simulink model "EGRVlv_VDPosGov"  (R2016b)
settings: configuration reference "CodeGenConfigSet" (kept outside this file)
values from neighbouring files (symbols this model uses):
  EGRVlv_ctClnUpFin_C = Calibration.Parameter    [init_EGRVlv_VDPosGov.m]
  EGRVlv_DKdNgv_C = Calibration.Parameter    [init_EGRVlv_VDPosGov.m]
  EGRVlv_DKdPsv_C = Calibration.Parameter    [init_EGRVlv_VDPosGov.m]
  EGRVlv_drActNgv_C = Calibration.Parameter    [init_EGRVlv_VDPosGov.m]
  EGRVlv_facCrntEffFlt_C = Calibration.Parameter    [init_EGRVlv_VDPosGov.m]
  EGRVlv_iEff_CUR = Calibration.Parameter    [init_EGRVlv_VDPosGov.m]
  EGRVlv_iEff_CURX = Calibration.Parameter    [init_EGRVlv_VDPosGov.m]
  EGRVlv_iEffOvrLd_C = Calibration.Parameter    [init_EGRVlv_VDPosGov.m]
  EGRVlv_IKiLMSSlp_C = Calibration.Parameter    [init_EGRVlv_VDPosGov.m]
  EGRVlv_IKiNgv_C = Calibration.Parameter    [init_EGRVlv_VDPosGov.m]
  EGRVlv_IKiPsv_C = Calibration.Parameter    [init_EGRVlv_VDPosGov.m]
  EGRVlv_KdParDT1_C = Calibration.Parameter    [init_EGRVlv_VDPosGov.m]
  EGRVlv_PKpNgv_C = Calibration.Parameter    [init_EGRVlv_VDPosGov.m]
  EGRVlv_PKpPsv_C = Calibration.Parameter    [init_EGRVlv_VDPosGov.m]
  EGRVlv_rActNgv_C = Calibration.Parameter    [init_EGRVlv_VDPosGov.m]
  EGRVlv_rDesClnUpCls_C = Calibration.Parameter    [init_EGRVlv_VDPosGov.m]
  EGRVlv_rDesClnUpOpen_C = Calibration.Parameter    [init_EGRVlv_VDPosGov.m]
  EGRVlv_rDesEGR_CUR = Calibration.Parameter    [init_EGRVlv_VDPosGov.m]
  EGRVlv_rDesEGR_CURX = Calibration.Parameter    [init_EGRVlv_VDPosGov.m]
  EGRVlv_rDesLMSMin_C = Calibration.Parameter    [init_EGRVlv_VDPosGov.m]
  EGRVlv_rDesOffHold_C = Calibration.Parameter    [init_EGRVlv_VDPosGov.m]
  EGRVlv_rEGRDflVal_C = Calibration.Parameter    [init_EGRVlv_VDPosGov.m]
  EGRVlv_rEGRSwtOff_C = Calibration.Parameter    [init_EGRVlv_VDPosGov.m]
  EGRVlv_rGovDvtThres_C = Calibration.Parameter    [init_EGRVlv_VDPosGov.m]
  EGRVlv_rGovMax_C = Calibration.Parameter    [init_EGRVlv_VDPosGov.m]
  EGRVlv_rGovMax_CUR = Calibration.Parameter    [init_EGRVlv_VDPosGov.m]
  EGRVlv_rGovMax_CURX = Calibration.Parameter    [init_EGRVlv_VDPosGov.m]
  EGRVlv_rGovMin_C = Calibration.Parameter    [init_EGRVlv_VDPosGov.m]
  EGRVlv_rGovMin_CUR = Calibration.Parameter    [init_EGRVlv_VDPosGov.m]
  EGRVlv_rGovMin_CURX = Calibration.Parameter    [init_EGRVlv_VDPosGov.m]
  EGRVlv_rIniStp_C = Calibration.Parameter    [init_EGRVlv_VDPosGov.m]
  EGRVlv_rOutDMax_C = Calibration.Parameter    [init_EGRVlv_VDPosGov.m]
  EGRVlv_rOutIMax_C = Calibration.Parameter    [init_EGRVlv_VDPosGov.m]
  EGRVlv_rPIDWinNgv_C = Calibration.Parameter    [init_EGRVlv_VDPosGov.m]
  EGRVlv_rPIDWinPsv_C = Calibration.Parameter    [init_EGRVlv_VDPosGov.m]
  EGRVlv_rSwtOffRmp_C = Calibration.Parameter    [init_EGRVlv_VDPosGov.m]
  EGRVlv_SlwClsDKd_C = Calibration.Parameter    [init_EGRVlv_VDPosGov.m]
  EGRVlv_SlwClsIKi_C = Calibration.Parameter    [init_EGRVlv_VDPosGov.m]
  EGRVlv_SlwClsPKp_C = Calibration.Parameter    [init_EGRVlv_VDPosGov.m]
  EGRVlv_SmlSigNgvDKd_C = Calibration.Parameter    [init_EGRVlv_VDPosGov.m]
  EGRVlv_SmlSigNgvIKi_C = Calibration.Parameter    [init_EGRVlv_VDPosGov.m]
  EGRVlv_SmlSigNgvPKp_C = Calibration.Parameter    [init_EGRVlv_VDPosGov.m]
  EGRVlv_SmlSigPsvDKd_C = Calibration.Parameter    [init_EGRVlv_VDPosGov.m]
  EGRVlv_SmlSigPsvIKi_C = Calibration.Parameter    [init_EGRVlv_VDPosGov.m]
  EGRVlv_SmlSigPsvPKp_C = Calibration.Parameter    [init_EGRVlv_VDPosGov.m]
  EGRVLV_STCLNUP_CLOSE = fi(3,State_uint8)    [init_EGRVlv_VDPosGov.m]
  EGRVLV_STCLNUP_FINISH = fi(4,State_uint8)    [init_EGRVlv_VDPosGov.m]
  EGRVLV_STCLNUP_INIT = fi(1,State_uint8)    [init_EGRVlv_VDPosGov.m]
  EGRVLV_STCLNUP_OPEN = fi(2,State_uint8)    [init_EGRVlv_VDPosGov.m]
  EGRVlv_stClnUpInh_C = Calibration.Parameter    [init_EGRVlv_VDPosGov.m]
  EGRVlv_swtDesValNrmInv_C = Calibration.Parameter    [init_EGRVlv_VDPosGov.m]
  EGRVlv_swtEGRTyp_C = Calibration.Parameter    [init_EGRVlv_VDPosGov.m]
  EGRVlv_swtGovByp_C = Calibration.Parameter    [init_EGRVlv_VDPosGov.m]
  EGRVlv_swtSelDT1In_C = Calibration.Parameter    [init_EGRVlv_VDPosGov.m]
  EGRVlv_tiClnUp_C = Calibration.Parameter    [init_EGRVlv_VDPosGov.m]
  EGRVlv_tiGovDT1_C = Calibration.Parameter    [init_EGRVlv_VDPosGov.m]
  EGRVlv_tiLimDlyOvrLd_C = Calibration.Parameter    [init_EGRVlv_VDPosGov.m]
  EGRVlv_tiOutIMax_C = Calibration.Parameter    [init_EGRVlv_VDPosGov.m]
  EGRVlv_tiParDT1_C = Calibration.Parameter    [init_EGRVlv_VDPosGov.m]
  MINUS_1_PRC = fi(-1,Prc_100_rate)    [init_EGRVlv_VDPosGov.m]
  RLS = fi(0,State_uint8)    [init_EGRVlv_VDPosGov.m]
  VALEO = fi(0,State_uint8)    [init_EGRVlv_VDPosGov.m]
  ZERO_PRC = fi(0,Prc_100_rate)    [init_EGRVlv_VDPosGov.m]
undefined symbols (not defined in the file or in its folder): CEngDsT_tTransf_CURX, EGRVlv_VDPosGov_DT, SubSysExeState_conv
libraries: CXLib x32, simulink x12
(part 1 of 2)
settings Model: Creator=lvzhanghui  LastModifiedBy=zhoutinglin
settings ConfigSetRef: SourceLocation=Base Workspace

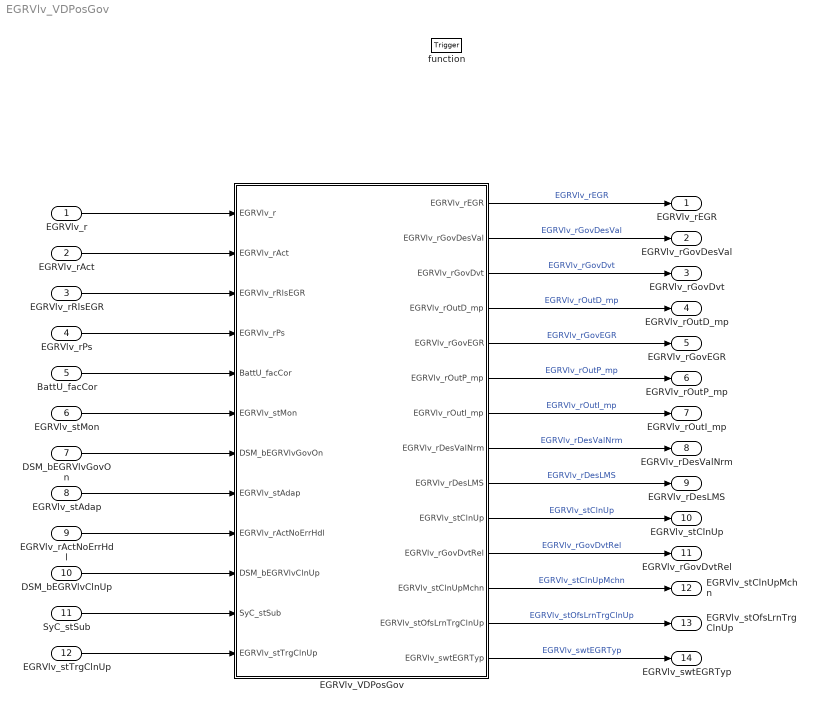
== system EGRVlv_VDPosGov ==
  EGRVlv_r : Inport  Tag=%  Description=Commanded value from application SW  OutMin=-100  OutMax=100  OutDataTypeStr=Prc_100_rate
  EGRVlv_rAct : Inport  Tag=%  Description=Actuatorposition  Port=2  OutMin=-100  OutMax=100  OutDataTypeStr=Prc_100_rate
  EGRVlv_rRlsEGR : Inport  Tag=%  Description=Additional control value to release a jammed valve  Port=3  OutMin=-100  OutMax=100  OutDataTypeStr=Prc_100_rate
  EGRVlv_rPs : Inport  Tag=%  Description=Duty cycle to power stage  Port=4  OutMin=-100  OutMax=100  OutDataTypeStr=Prc_100_rate
  BattU_facCor : Inport  Description=Battery correction factor  Port=5  OutMin=-32  OutMax=31.9  OutDataTypeStr=Factor
  EGRVlv_stMon : Inport  Description=State of system monitoring  Port=6  OutMin=0  OutMax=65535  OutDataTypeStr=State_uint16
  DSM_bEGRVlvGovOn : Inport  Description=Status of FId_EGRVlvGovOn  Port=7  OutMin=0  OutMax=1  OutDataTypeStr=boolean
  EGRVlv_stAdap : Inport  Description=Status of offset learning  Port=8  OutMin=0  OutMax=65535  OutDataTypeStr=State_uint16
  EGRVlv_rActNoErrHdl : Inport  Tag=%  Description=Valve position (offset corrected without error handling)  Port=9  OutMin=-100  OutMax=100  OutDataTypeStr=Prc_100_rate
  DSM_bEGRVlvClnUp : Inport  Description=Status of FId_EGRVlvClnUp  Port=10  OutMin=0  OutMax=1  OutDataTypeStr=boolean
  SyC_stSub : Inport  Description=Current system/ECU sub-state  Port=11  OutDataTypeStr=Enum: SubSysExeState_conv
  EGRVlv_stTrgClnUp : Inport  Description=Status of valve cleaning trigger, in case of unsuccessful offset learning because of plausibility errors  Port=12  OutMin=0  OutMax=1  OutDataTypeStr=boolean
  function : TriggerPort  TriggerType=function-call  VariantControl=Variant
  EGRVlv_VDPosGov : Subsystem
  EGRVlv_rEGR : Outport  Tag=%  Description=Control value for the EGR valve  OutMin=-100  OutMax=100  OutDataTypeStr=Prc_100_rate
  EGRVlv_rGovDesVal : Outport  Tag=%  Description=Internal desired value for governor  Port=2  OutMin=-100  OutMax=100  OutDataTypeStr=Prc_100_rate
  EGRVlv_rGovDvt : Outport  Tag=%  Description=Control deviation  Port=3  OutMin=-100  OutMax=100  OutDataTypeStr=Prc_100_rate
  EGRVlv_rOutD_mp : Outport  Tag=%  Description=measurement point for D governor for single flow implementation  Port=4  OutMin=-100  OutMax=100  OutDataTypeStr=Prc_100_rate
  EGRVlv_rGovEGR : Outport  Tag=%  Description=Control value from the governor  Port=5  OutMin=-100  OutMax=100  OutDataTypeStr=Prc_100_rate
  EGRVlv_rOutP_mp : Outport  Tag=%  Description=measurement point for P governor for single flow implementation  Port=6  OutMin=-100  OutMax=100  OutDataTypeStr=Prc_100_rate
  EGRVlv_rOutI_mp : Outport  Tag=%  Description=measurement point for I governor for single flow implementation  Port=7  OutMin=-100  OutMax=100  OutDataTypeStr=Prc_100_rate
  EGRVlv_rDesValNrm : Outport  Tag=%  Description=Normalized desired value  Port=8  OutMin=-100  OutMax=100  OutDataTypeStr=Prc_100_rate
  EGRVlv_rDesLMS : Outport  Tag=%  Description=Desired value from LMS control  Port=9  OutMin=-100  OutMax=100  OutDataTypeStr=Prc_100_rate
  EGRVlv_stClnUp : Outport  Description=Status of valvle cleanup function  Port=10  OutMin=0  OutMax=255  OutDataTypeStr=State_uint8
  EGRVlv_rGovDvtRel : Outport  Tag=%  Description=Relative governor deviation for OBD purpose  Port=11  OutMin=-100  OutMax=100  OutDataTypeStr=Prc_100_rate
  EGRVlv_stClnUpMchn : Outport  Description=Status of cleanup state machine  Port=12  OutMin=0  OutMax=255  OutDataTypeStr=State_uint8
  EGRVlv_stOfsLrnTrgClnUp : Outport  Description=Offset learning trigger from EGR valve cleanup function  Port=13  OutMin=0  OutMax=1  OutDataTypeStr=boolean
  EGRVlv_swtEGRTyp : Outport  Description=Type of EGR actuator used  Port=14  OutMin=0  OutMax=255  OutDataTypeStr=State_uint8
  wires:
  EGRVlv_r/1 -> EGRVlv_VDPosGov/1(EGRVlv_r)
  EGRVlv_rAct/1 -> EGRVlv_VDPosGov/2(EGRVlv_rAct)
  EGRVlv_rRlsEGR/1 -> EGRVlv_VDPosGov/3(EGRVlv_rRlsEGR)
  EGRVlv_rPs/1 -> EGRVlv_VDPosGov/4(EGRVlv_rPs)
  BattU_facCor/1 -> EGRVlv_VDPosGov/5(BattU_facCor)
  EGRVlv_stMon/1 -> EGRVlv_VDPosGov/6(EGRVlv_stMon)
  DSM_bEGRVlvGovOn/1 -> EGRVlv_VDPosGov/7(DSM_bEGRVlvGovOn)
  EGRVlv_stAdap/1 -> EGRVlv_VDPosGov/8(EGRVlv_stAdap)
  EGRVlv_rActNoErrHdl/1 -> EGRVlv_VDPosGov/9(EGRVlv_rActNoErrHdl)
  DSM_bEGRVlvClnUp/1 -> EGRVlv_VDPosGov/10(DSM_bEGRVlvClnUp)
  SyC_stSub/1 -> EGRVlv_VDPosGov/11(SyC_stSub)
  EGRVlv_stTrgClnUp/1 -> EGRVlv_VDPosGov/12(EGRVlv_stTrgClnUp)
  EGRVlv_VDPosGov/1(EGRVlv_rEGR) -> EGRVlv_rEGR/1  "EGRVlv_rEGR"
  EGRVlv_VDPosGov/2(EGRVlv_rGovDesVal) -> EGRVlv_rGovDesVal/1  "EGRVlv_rGovDesVal"
  EGRVlv_VDPosGov/3(EGRVlv_rGovDvt) -> EGRVlv_rGovDvt/1  "EGRVlv_rGovDvt"
  EGRVlv_VDPosGov/4(EGRVlv_rOutD_mp) -> EGRVlv_rOutD_mp/1  "EGRVlv_rOutD_mp"
  EGRVlv_VDPosGov/5(EGRVlv_rGovEGR) -> EGRVlv_rGovEGR/1  "EGRVlv_rGovEGR"
  EGRVlv_VDPosGov/6(EGRVlv_rOutP_mp) -> EGRVlv_rOutP_mp/1  "EGRVlv_rOutP_mp"
  EGRVlv_VDPosGov/7(EGRVlv_rOutI_mp) -> EGRVlv_rOutI_mp/1  "EGRVlv_rOutI_mp"
  EGRVlv_VDPosGov/8(EGRVlv_rDesValNrm) -> EGRVlv_rDesValNrm/1  "EGRVlv_rDesValNrm"
  EGRVlv_VDPosGov/9(EGRVlv_rDesLMS) -> EGRVlv_rDesLMS/1  "EGRVlv_rDesLMS"
  EGRVlv_VDPosGov/10(EGRVlv_stClnUp) -> EGRVlv_stClnUp/1  "EGRVlv_stClnUp"
  EGRVlv_VDPosGov/11(EGRVlv_rGovDvtRel) -> EGRVlv_rGovDvtRel/1  "EGRVlv_rGovDvtRel"
  EGRVlv_VDPosGov/12(EGRVlv_stClnUpMchn) -> EGRVlv_stClnUpMchn/1  "EGRVlv_stClnUpMchn"
  EGRVlv_VDPosGov/13(EGRVlv_stOfsLrnTrgClnUp) -> EGRVlv_stOfsLrnTrgClnUp/1  "EGRVlv_stOfsLrnTrgClnUp"
  EGRVlv_VDPosGov/14(EGRVlv_swtEGRTyp) -> EGRVlv_swtEGRTyp/1  "EGRVlv_swtEGRTyp"

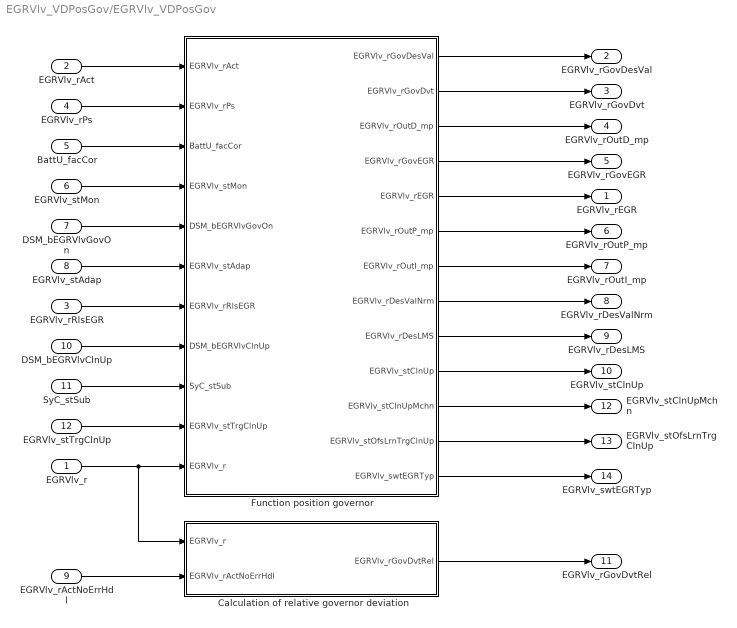
== system EGRVlv_VDPosGov/EGRVlv_VDPosGov ==
  EGRVlv_r : Inport  Tag=%
  EGRVlv_rAct : Inport  Tag=%  Port=2
  EGRVlv_rRlsEGR : Inport  Tag=%  Port=3
  EGRVlv_rPs : Inport  Tag=%  Port=4
  BattU_facCor : Inport  Port=5
  EGRVlv_stMon : Inport  Port=6
  DSM_bEGRVlvGovOn : Inport  Port=7
  EGRVlv_stAdap : Inport  Port=8
  EGRVlv_rActNoErrHdl : Inport  Tag=%  Port=9
  DSM_bEGRVlvClnUp : Inport  Tag=%  Port=10
  SyC_stSub : Inport  Tag=%  Port=11
  EGRVlv_stTrgClnUp : Inport  Tag=%  Port=12
  Calculation of relative governor deviation : Subsystem
  Function position governor : Subsystem
  EGRVlv_rEGR : Outport  Tag=%
  EGRVlv_rGovDesVal : Outport  Tag=%  Port=2
  EGRVlv_rGovDvt : Outport  Tag=%  Port=3
  EGRVlv_rOutD_mp : Outport  Tag=%  Port=4
  EGRVlv_rGovEGR : Outport  Tag=%  Port=5
  EGRVlv_rOutP_mp : Outport  Tag=%  Port=6
  EGRVlv_rOutI_mp : Outport  Tag=%  Port=7
  EGRVlv_rDesValNrm : Outport  Tag=%  Port=8
  EGRVlv_rDesLMS : Outport  Tag=%  Port=9
  EGRVlv_stClnUp : Outport  Port=10
  EGRVlv_rGovDvtRel : Outport  Tag=%  Port=11
  EGRVlv_stClnUpMchn : Outport  Tag=%  Port=12
  EGRVlv_stOfsLrnTrgClnUp : Outport  Tag=%  Port=13
  EGRVlv_swtEGRTyp : Outport  Tag=%  Port=14
  wires:
  EGRVlv_r/1 -> Function position governor/11(EGRVlv_r), Calculation of relative governor deviation/1(EGRVlv_r)
  EGRVlv_rActNoErrHdl/1 -> Calculation of relative governor deviation/2(EGRVlv_rActNoErrHdl)
  EGRVlv_rAct/1 -> Function position governor/1(EGRVlv_rAct)
  EGRVlv_rPs/1 -> Function position governor/2(EGRVlv_rPs)
  BattU_facCor/1 -> Function position governor/3(BattU_facCor)
  EGRVlv_stMon/1 -> Function position governor/4(EGRVlv_stMon)
  DSM_bEGRVlvGovOn/1 -> Function position governor/5(DSM_bEGRVlvGovOn)
  EGRVlv_stAdap/1 -> Function position governor/6(EGRVlv_stAdap)
  EGRVlv_rRlsEGR/1 -> Function position governor/7(EGRVlv_rRlsEGR)
  DSM_bEGRVlvClnUp/1 -> Function position governor/8(DSM_bEGRVlvClnUp)
  SyC_stSub/1 -> Function position governor/9(SyC_stSub)
  EGRVlv_stTrgClnUp/1 -> Function position governor/10(EGRVlv_stTrgClnUp)
  Calculation of relative governor deviation/1(EGRVlv_rGovDvtRel) -> EGRVlv_rGovDvtRel/1
  Function position governor/1(EGRVlv_rGovDesVal) -> EGRVlv_rGovDesVal/1
  Function position governor/2(EGRVlv_rGovDvt) -> EGRVlv_rGovDvt/1
  Function position governor/3(EGRVlv_rOutD_mp) -> EGRVlv_rOutD_mp/1
  Function position governor/4(EGRVlv_rGovEGR) -> EGRVlv_rGovEGR/1
  Function position governor/5(EGRVlv_rEGR) -> EGRVlv_rEGR/1
  Function position governor/6(EGRVlv_rOutP_mp) -> EGRVlv_rOutP_mp/1
  Function position governor/7(EGRVlv_rOutI_mp) -> EGRVlv_rOutI_mp/1
  Function position governor/8(EGRVlv_rDesValNrm) -> EGRVlv_rDesValNrm/1
  Function position governor/9(EGRVlv_rDesLMS) -> EGRVlv_rDesLMS/1
  Function position governor/10(EGRVlv_stClnUp) -> EGRVlv_stClnUp/1
  Function position governor/11(EGRVlv_stClnUpMchn) -> EGRVlv_stClnUpMchn/1
  Function position governor/12(EGRVlv_stOfsLrnTrgClnUp) -> EGRVlv_stOfsLrnTrgClnUp/1
  Function position governor/13(EGRVlv_swtEGRTyp) -> EGRVlv_swtEGRTyp/1

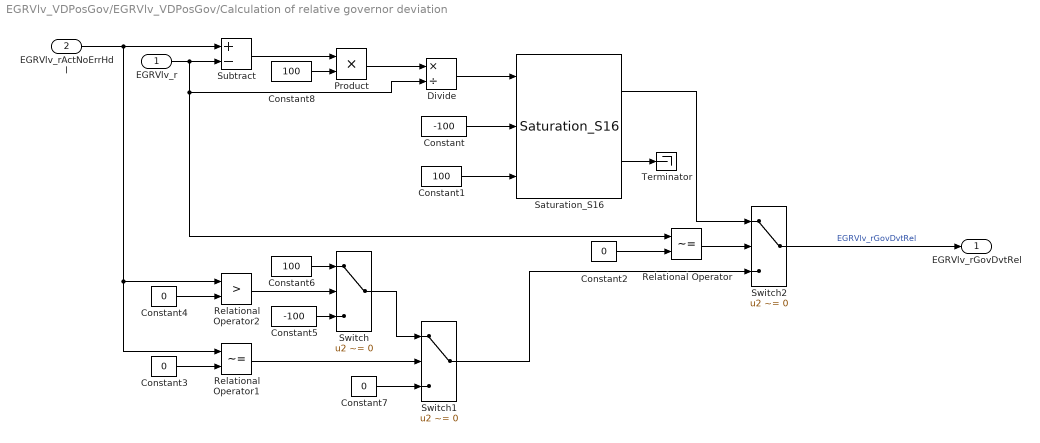
== system EGRVlv_VDPosGov/EGRVlv_VDPosGov/Calculation of relative governor deviation ==
  EGRVlv_r : Inport  Tag=%
  EGRVlv_rActNoErrHdl : Inport  Tag=%  Port=2
  Constant : Constant  Value=-100  OutDataTypeStr=Prc_100_rate
  Constant1 : Constant  Value=100  OutDataTypeStr=Prc_100_rate
  Constant2 : Constant  Value=0  OutDataTypeStr=Inherit: Inherit via back propagation
  Constant3 : Constant  Value=0  OutDataTypeStr=Inherit: Inherit via back propagation
  Constant4 : Constant  Value=0  OutDataTypeStr=Inherit: Inherit via back propagation
  Constant5 : Constant  Value=-100  OutDataTypeStr=Prc_100_rate
  Constant6 : Constant  Value=100  OutDataTypeStr=Prc_100_rate
  Constant7 : Constant  Value=0  OutDataTypeStr=Prc_100_rate
  Constant8 : Constant  Value=100  OutDataTypeStr=uint8
  Divide : Product  Inputs=*/  OutDataTypeStr=Prc_100_rate  SaturateOnIntegerOverflow=on
  Product : Product  OutDataTypeStr=fixdt(1,16,10000/8192,0)  SaturateOnIntegerOverflow=on
  Relational Operator : RelationalOperator  Operator=~=  OutDataTypeStr=boolean  RndMeth=Simplest  InputSameDT=on
  Relational Operator1 : RelationalOperator  Operator=~=  OutDataTypeStr=boolean  RndMeth=Simplest  InputSameDT=on
  Relational Operator2 : RelationalOperator  Operator=>  OutDataTypeStr=boolean  RndMeth=Simplest  InputSameDT=on
  Saturation_S16 : CXLib/Saturation_S16
  Subtract : Sum  Inputs=+-  SaturateOnIntegerOverflow=on
  Switch : Switch  Criteria=u2 ~= 0
  Switch1 : Switch  Criteria=u2 ~= 0
  Switch2 : Switch  Criteria=u2 ~= 0
  Terminator : Terminator
  EGRVlv_rGovDvtRel : Outport  Tag=%
  wires:
  EGRVlv_r/1 -> Relational Operator/1, Divide/2, Subtract/2
  Subtract/1 -> Product/1
  Product/1 -> Divide/1
  Divide/1 -> Saturation_S16/1
  Constant/1 -> Saturation_S16/2
  Constant1/1 -> Saturation_S16/3
  Constant2/1 -> Relational Operator/2
  EGRVlv_rActNoErrHdl/1 -> Subtract/1, Relational Operator1/1, Relational Operator2/1
  Constant3/1 -> Relational Operator1/2
  Constant4/1 -> Relational Operator2/2
  Relational Operator2/1 -> Switch/2
  Constant6/1 -> Switch/1
  Constant5/1 -> Switch/3
  Switch/1 -> Switch1/1
  Constant7/1 -> Switch1/3
  Relational Operator1/1 -> Switch1/2
  Relational Operator/1 -> Switch2/2
  Switch1/1 -> Switch2/3
  Saturation_S16/1 -> Switch2/1
  Switch2/1 -> EGRVlv_rGovDvtRel/1  "EGRVlv_rGovDvtRel"
  Constant8/1 -> Product/2
  Saturation_S16/2 -> Terminator/1

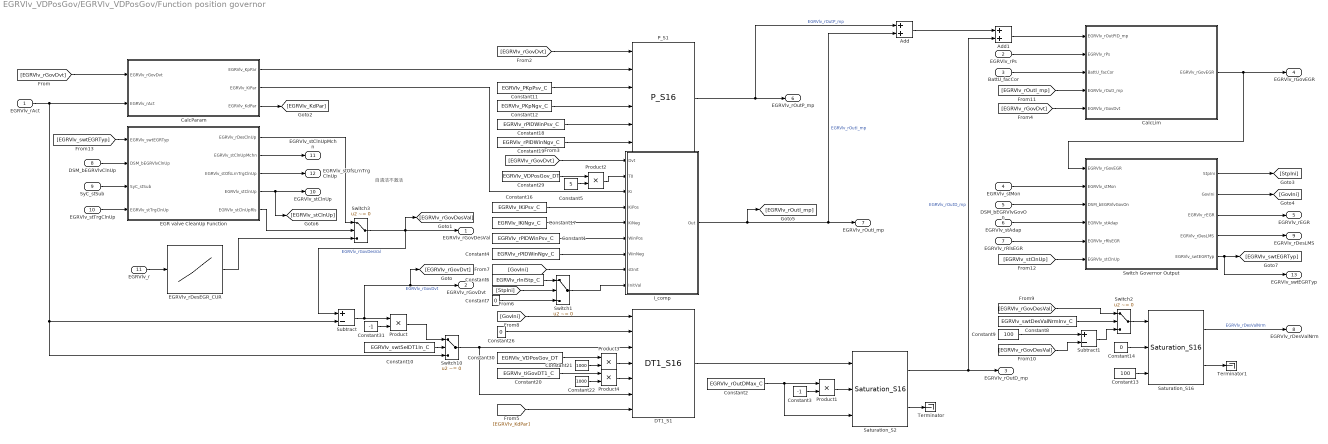
== system EGRVlv_VDPosGov/EGRVlv_VDPosGov/Function position governor ==
  note: 自清洁不激活
  EGRVlv_rAct : Inport  Tag=%
  EGRVlv_rPs : Inport  Tag=%  Port=2
  BattU_facCor : Inport  Tag=%  Port=3
  EGRVlv_stMon : Inport  Tag=%  Port=4
  DSM_bEGRVlvGovOn : Inport  Tag=%  Port=5
  EGRVlv_stAdap : Inport  Tag=%  Port=6
  EGRVlv_rRlsEGR : Inport  Tag=%  Port=7
  DSM_bEGRVlvClnUp : Inport  Tag=%  Port=8
  SyC_stSub : Inport  Tag=%  Port=9
  EGRVlv_stTrgClnUp : Inport  Tag=%  Port=10
  EGRVlv_r : Inport  Tag=%  Port=11
  Add : Sum  SaturateOnIntegerOverflow=on
  Add1 : Sum  SaturateOnIntegerOverflow=on
  CalcLim : Subsystem
  CalcParam : Subsystem
  Constant1 : Constant  Value=EGRVlv_rPIDWinPsv_C
  Constant10 : Constant  Value=EGRVlv_swtSelDT1In_C
  Constant11 : Constant  Value=EGRVlv_PKpPsv_C
  Constant12 : Constant  Value=EGRVlv_PKpNgv_C
  Constant13 : Constant  Value=100  OutDataTypeStr=Prc_100_rate
  Constant14 : Constant  Value=0  OutDataTypeStr=Prc_100_rate
  Constant16 : Constant  Value=EGRVlv_IKiPsv_C
  Constant17 : Constant  Value=EGRVlv_IKiNgv_C
  Constant18 : Constant  Value=EGRVlv_rPIDWinPsv_C
  Constant19 : Constant  Value=EGRVlv_rPIDWinNgv_C
  Constant2 : Constant  Value=EGRVlv_rOutDMax_C
  Constant20 : Constant  Value=EGRVlv_tiGovDT1_C
  Constant21 : Constant  Value=1000  OutDataTypeStr=uint16
  Constant22 : Constant  Value=1000  OutDataTypeStr=uint16
  Constant26 : Constant  Value=0  OutDataTypeStr=Inherit: Inherit via back propagation
  Constant29 : Constant  Value=EGRVlv_VDPosGov_DT
  Constant3 : Constant  Value=-1  OutDataTypeStr=int8
  Constant30 : Constant  Value=EGRVlv_VDPosGov_DT
  Constant31 : Constant  Value=-1  OutDataTypeStr=int8
  Constant4 : Constant  Value=EGRVlv_rPIDWinNgv_C
  Constant5 : Constant  Value=5  OutDataTypeStr=uint32
  Constant6 : Constant  Value=EGRVlv_rIniStp_C
  Constant7 : Constant  Value=0  OutDataTypeStr=Inherit: Inherit via back propagation
  Constant8 : Constant  Value=EGRVlv_swtDesValNrmInv_C
  Constant9 : Constant  Value=100  OutDataTypeStr=Prc_100_rate
  DT1_S1 : CXLib/DT1_S16
  EGR valve CleanUp Function : Subsystem
  EGRVlv_rDesEGR_CUR : Lookup_n-D  DialogController=Simulink.DDGSource  NumberOfTableDimensions=1  BreakpointsForDimension1=EGRVlv_rDesEGR_CURX  BreakpointsForDimension2=CEngDsT_tTransf_CURX  IndexSearchMethod=Linear search  BeginIndexSearchUsingPreviousIndexResult=on  Table=EGRVlv_rDesEGR_CUR  TableDataTypeStr=Inherit: Inherit from 'Table data'  ExtrapMethod=Clip  UseLastTableValue=on  InternalRulePriority=Speed  OutDataTypeStr=Inherit: Inherit from 'Table data'  SaturateOnIntegerOverflow=on
  I_comp : Subsystem
  P_S1 : CXLib/P_S16
  Product : Product  OutDataTypeStr=Prc_100_rate  SaturateOnIntegerOverflow=on
  Product1 : Product  OutDataTypeStr=Prc_100_rate  SaturateOnIntegerOverflow=on
  Product2 : Product  OutDataTypeStr=Inherit: Inherit via back propagation  SaturateOnIntegerOverflow=on
  Product3 : Product  OutDataTypeStr=uint32  SaturateOnIntegerOverflow=on
  Product4 : Product  OutDataTypeStr=uint32  SaturateOnIntegerOverflow=on
  Saturation_S16 : CXLib/Saturation_S16
  Saturation_S2 : CXLib/Saturation_S16
  Subtract : Sum  Inputs=+-  SaturateOnIntegerOverflow=on
  Subtract1 : Sum  Inputs=+-  SaturateOnIntegerOverflow=on
  Switch Governor Output : Subsystem
  Switch{1..3,10} (4 alike) : Switch  Criteria=u2 ~= 0
  Terminator : Terminator
  Terminator1 : Terminator
  EGRVlv_rGovDesVal : Outport  Tag=%
  EGRVlv_rGovDvt : Outport  Tag=%  Port=2
  EGRVlv_rOutD_mp : Outport  Tag=%  Port=3
  EGRVlv_rGovEGR : Outport  Tag=%  Port=4
  EGRVlv_rEGR : Outport  Tag=%  Port=5
  EGRVlv_rOutP_mp : Outport  Tag=%  Port=6
  EGRVlv_rOutI_mp : Outport  Tag=%  Port=7
  EGRVlv_rDesValNrm : Outport  Tag=%  Port=8
  EGRVlv_rDesLMS : Outport  Tag=%  Port=9
  EGRVlv_stClnUp : Outport  Tag=%  Port=10
  EGRVlv_stClnUpMchn : Outport  Tag=%  Port=11
  EGRVlv_stOfsLrnTrgClnUp : Outport  Tag=%  Port=12
  EGRVlv_swtEGRTyp : Outport  Tag=%  Port=13
  wires:
  Constant7/1 -> Switch1/3
  Constant8/1 -> Switch2/2
  Constant9/1 -> Subtract1/1
  EGRVlv_r/1 -> EGRVlv_rDesEGR_CUR/1
  Switch3/1 -> [EGRVlv_rGovDesVal], EGRVlv_rGovDesVal/1, Subtract/1  "EGRVlv_rGovDesVal"
  EGRVlv_rAct/1 -> CalcParam/2(EGRVlv_rAct), Subtract/2, Switch10/3
  Switch10/1 -> DT1_S1/6, DT1_S1/3
  Constant26/1 -> DT1_S1/2
  Constant10/1 -> Switch10/2
  Subtract/1 -> EGRVlv_rGovDvt/1, [EGRVlv_rGovDvt], Product/1  "EGRVlv_rGovDvt"
  Constant31/1 -> Product/2
  Product/1 -> Switch10/1
  DT1_S1/1 -> Saturation_S2/1
  Constant2/1 -> Saturation_S2/3, Product1/1
  Constant3/1 -> Product1/2
  Product1/1 -> Saturation_S2/2
  Saturation_S2/1 -> EGRVlv_rOutD_mp/1, Add1/2  "EGRVlv_rOutD_mp"
  Add/1 -> Add1/1
  Add1/1 -> CalcLim/1(EGRVlv_rOutPID_mp)
  [StpIni] -> Switch1/2
  Constant6/1 -> Switch1/1
  [EGRVlv_rGovDesVal] -> Subtract1/2
  Subtract1/1 -> Switch2/3
  [EGRVlv_rGovDesVal] -> Switch2/1
  Switch1/1 -> I_comp/9(InitVal)
  Constant14/1 -> Saturation_S16/2
  Constant12/1 -> P_S1/4
  Constant1/1 -> I_comp/6(WinPos)
  P_S1/1 -> EGRVlv_rOutP_mp/1, Add/1  "EGRVlv_rOutP_mp"
  Constant4/1 -> I_comp/7(WinNeg)
  Constant11/1 -> P_S1/3
  Constant19/1 -> P_S1/6
  Constant16/1 -> I_comp/4(KiPos)
  CalcParam/1(EGRVlv_KpPar) -> P_S1/2
  Constant18/1 -> P_S1/5
  CalcParam/2(EGRVlv_KiPar) -> I_comp/3(Ki)
  Constant17/1 -> I_comp/5(KiNeg)
  I_comp/1(Out) -> EGRVlv_rOutI_mp/1, Add/2, [EGRVlv_rOutI_mp]  "EGRVlv_rOutI_mp"
  CalcLim/1(EGRVlv_rGovEGR) -> EGRVlv_rGovEGR/1, Switch Governor Output/1(EGRVlv_rGovEGR)
  Constant13/1 -> Saturation_S16/3
  Switch2/1 -> Saturation_S16/1
  EGRVlv_rDesEGR_CUR/1 -> Switch3/3
  EGR valve CleanUp Function/1(EGRVlv_rDesClnUp) -> Switch3/1
  Constant21/1 -> Product3/2
  Product3/1 -> DT1_S1/4
  Constant30/1 -> Product3/1
  Constant22/1 -> Product4/2
  Constant20/1 -> Product4/1
  Product4/1 -> DT1_S1/5
  Switch Governor Output/5(EGRVlv_swtEGRTyp) -> EGRVlv_swtEGRTyp/1, [EGRVlv_swtEGRTyp]
  EGR valve CleanUp Function/4(EGRVlv_stClnUp) -> [EGRVlv_stClnUp], EGRVlv_stClnUp/1
  EGR valve CleanUp Function/5(EGRVlv_stClnUpRls) -> Switch3/2
  EGRVlv_rPs/1 -> CalcLim/2(EGRVlv_rPs)
  BattU_facCor/1 -> CalcLim/3(BattU_facCor)
  [EGRVlv_rOutI_mp] -> CalcLim/4(EGRVlv_rOutI_mp)
  [EGRVlv_rGovDvt] -> CalcParam/1(EGRVlv_rGovDvt)
  [GovIni] -> DT1_S1/1
  [EGRVlv_KdPar] -> DT1_S1/7
  [EGRVlv_swtEGRTyp] -> EGR valve CleanUp Function/1(EGRVlv_swtEGRTyp)
  DSM_bEGRVlvClnUp/1 -> EGR valve CleanUp Function/2(DSM_bEGRVlvClnUp)
  SyC_stSub/1 -> EGR valve CleanUp Function/3(SyC_stSub)
  EGRVlv_stTrgClnUp/1 -> EGR valve CleanUp Function/4(EGRVlv_stTrgClnUp)
  [EGRVlv_rGovDvt] -> I_comp/1(Dvt)
  [GovIni] -> I_comp/8(stInit)
  [EGRVlv_rGovDvt] -> CalcLim/5(EGRVlv_rGovDvt)
  [EGRVlv_rGovDvt] -> P_S1/1
  EGRVlv_stMon/1 -> Switch Governor Output/2(EGRVlv_stMon)
  DSM_bEGRVlvGovOn/1 -> Switch Governor Output/3(DSM_bEGRVlvGovOn)
  EGRVlv_stAdap/1 -> Switch Governor Output/4(EGRVlv_stAdap)
  EGRVlv_rRlsEGR/1 -> Switch Governor Output/5(EGRVlv_rRlsEGR)
  [EGRVlv_stClnUp] -> Switch Governor Output/6(EGRVlv_stClnUp)
  CalcParam/3(EGRVlv_KdPar) -> [EGRVlv_KdPar]
  EGR valve CleanUp Function/2(EGRVlv_stClnUpMchn) -> EGRVlv_stClnUpMchn/1
  EGR valve CleanUp Function/3(EGRVlv_stOfsLrnTrgClnUp) -> EGRVlv_stOfsLrnTrgClnUp/1
  Saturation_S16/1 -> EGRVlv_rDesValNrm/1  "EGRVlv_rDesValNrm"
  Saturation_S16/2 -> Terminator1/1
  Saturation_S2/2 -> Terminator/1
  Switch Governor Output/1(StpIni) -> [StpIni]
  Switch Governor Output/2(GovIni) -> [GovIni]
  Switch Governor Output/3(EGRVlv_rEGR) -> EGRVlv_rEGR/1
  Switch Governor Output/4(EGRVlv_rDesLMS) -> EGRVlv_rDesLMS/1
  Constant29/1 -> Product2/1
  Product2/1 -> I_comp/2(T0)
  Constant5/1 -> Product2/2

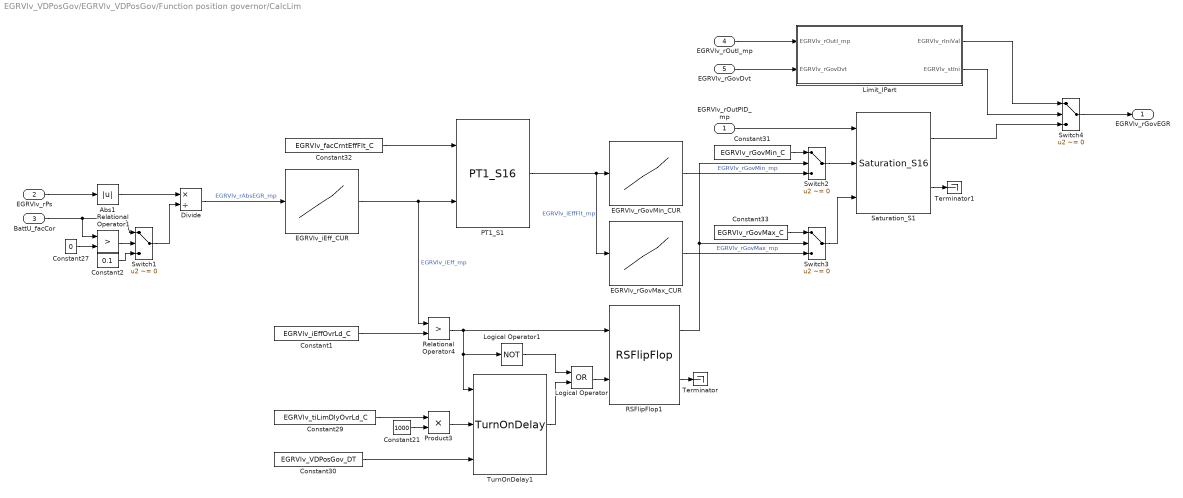
== system EGRVlv_VDPosGov/EGRVlv_VDPosGov/Function position governor/CalcLim ==
  EGRVlv_rOutPID_mp : Inport  Tag=%
  EGRVlv_rPs : Inport  Tag=%  Port=2
  BattU_facCor : Inport  Tag=%  Port=3
  EGRVlv_rOutI_mp : Inport  Tag=%  Port=4
  EGRVlv_rGovDvt : Inport  Tag=%  Port=5
  Abs1 : Abs
  Constant1 : Constant  Value=EGRVlv_iEffOvrLd_C
  Constant2 : Constant  Value=0.1  OutDataTypeStr=Inherit: Inherit via back propagation
  Constant21 : Constant  Value=1000  OutDataTypeStr=uint16
  Constant27 : Constant  Value=0  OutDataTypeStr=Inherit: Inherit via back propagation
  Constant29 : Constant  Value=EGRVlv_tiLimDlyOvrLd_C
  Constant30 : Constant  Value=EGRVlv_VDPosGov_DT
  Constant31 : Constant  Value=EGRVlv_rGovMin_C
  Constant32 : Constant  Value=EGRVlv_facCrntEffFlt_C
  Constant33 : Constant  Value=EGRVlv_rGovMax_C
  Divide : Product  Inputs=*/  OutDataTypeStr=Prc_100_rate  SaturateOnIntegerOverflow=on
  EGRVlv_iEff_CUR : Lookup_n-D  DialogController=Simulink.DDGSource  NumberOfTableDimensions=1  BreakpointsForDimension1=EGRVlv_iEff_CURX  BreakpointsForDimension2=CEngDsT_tTransf_CURX  IndexSearchMethod=Linear search  BeginIndexSearchUsingPreviousIndexResult=on  Table=EGRVlv_iEff_CUR  TableDataTypeStr=Inherit: Inherit from 'Table data'  ExtrapMethod=Clip  UseLastTableValue=on  InternalRulePriority=Speed  OutDataTypeStr=Inherit: Inherit from 'Table data'  SaturateOnIntegerOverflow=on
  EGRVlv_rGovMax_CUR : Lookup_n-D  DialogController=Simulink.DDGSource  NumberOfTableDimensions=1  BreakpointsForDimension1=EGRVlv_rGovMax_CURX  BreakpointsForDimension2=CEngDsT_tTransf_CURX  IndexSearchMethod=Linear search  BeginIndexSearchUsingPreviousIndexResult=on  Table=EGRVlv_rGovMax_CUR  TableDataTypeStr=Inherit: Inherit from 'Table data'  ExtrapMethod=Clip  UseLastTableValue=on  InternalRulePriority=Speed  OutDataTypeStr=Inherit: Inherit from 'Table data'  SaturateOnIntegerOverflow=on
  EGRVlv_rGovMin_CUR : Lookup_n-D  DialogController=Simulink.DDGSource  NumberOfTableDimensions=1  BreakpointsForDimension1=EGRVlv_rGovMin_CURX  BreakpointsForDimension2=CEngDsT_tTransf_CURX  IndexSearchMethod=Linear search  BeginIndexSearchUsingPreviousIndexResult=on  Table=EGRVlv_rGovMin_CUR  TableDataTypeStr=Inherit: Inherit from 'Table data'  ExtrapMethod=Clip  UseLastTableValue=on  InternalRulePriority=Speed  OutDataTypeStr=Inherit: Inherit from 'Table data'  SaturateOnIntegerOverflow=on
  Limit_IPart : Subsystem
  Logical Operator : Logic  Operator=OR  AllPortsSameDT=off  OutDataTypeStr=boolean
  Logical Operator1 : Logic  Operator=NOT  AllPortsSameDT=off  OutDataTypeStr=boolean
  PT1_S1 : CXLib/PT1_S16
  Product3 : Product  OutDataTypeStr=uint32  SaturateOnIntegerOverflow=on
  RSFlipFlop1 : CXLib/RSFlipFlop
  Relational Operator1 : RelationalOperator  Operator=>  OutDataTypeStr=boolean  RndMeth=Simplest  InputSameDT=on
  Relational Operator4 : RelationalOperator  Operator=>  OutDataTypeStr=boolean  RndMeth=Simplest
  Saturation_S1 : CXLib/Saturation_S16
  Switch{1..4} (4 alike) : Switch  Criteria=u2 ~= 0
  Terminator : Terminator
  Terminator1 : Terminator
  TurnOnDelay1 : CXLib/TurnOnDelay
  EGRVlv_rGovEGR : Outport  Tag=%
  wires:
  Abs1/1 -> Divide/1
  Constant33/1 -> Switch3/1
  RSFlipFlop1/1 -> Switch3/2, Switch2/2
  EGRVlv_rGovMax_CUR/1 -> Switch3/3  "EGRVlv_rGovMax_mp"
  Switch2/1 -> Saturation_S1/2
  Switch3/1 -> Saturation_S1/3
  TurnOnDelay1/1 -> Logical Operator/2
  Logical Operator/1 -> RSFlipFlop1/2
  Logical Operator1/1 -> Logical Operator/1
  Constant31/1 -> Switch2/1
  EGRVlv_iEff_CUR/1 -> PT1_S1/2, Relational Operator4/1  "EGRVlv_iEff_mp"
  EGRVlv_rGovMin_CUR/1 -> Switch2/3  "EGRVlv_rGovMin_mp"
  Constant1/1 -> Relational Operator4/2
  Relational Operator4/1 -> RSFlipFlop1/1, TurnOnDelay1/1, Logical Operator1/1
  EGRVlv_rPs/1 -> Abs1/1
  Divide/1 -> EGRVlv_iEff_CUR/1  "EGRVlv_rAbsEGR_mp"
  PT1_S1/1 -> EGRVlv_rGovMax_CUR/1, EGRVlv_rGovMin_CUR/1  "EGRVlv_iEffFlt_mp"
  Constant29/1 -> Product3/1
  Constant30/1 -> TurnOnDelay1/3
  BattU_facCor/1 -> Relational Operator1/1, Switch1/1
  Constant32/1 -> PT1_S1/1
  Relational Operator1/1 -> Switch1/2
  Constant27/1 -> Relational Operator1/2
  Constant2/1 -> Switch1/3
  Switch1/1 -> Divide/2
  Product3/1 -> TurnOnDelay1/2
  Limit_IPart/1(EGRVlv_rIniVal) -> Switch4/1
  Limit_IPart/2(EGRVlv_stIni) -> Switch4/2
  Switch4/1 -> EGRVlv_rGovEGR/1
  Saturation_S1/1 -> Switch4/3
  Constant21/1 -> Product3/2
  EGRVlv_rOutPID_mp/1 -> Saturation_S1/1
  RSFlipFlop1/2 -> Terminator/1
  Saturation_S1/2 -> Terminator1/1
  EGRVlv_rGovDvt/1 -> Limit_IPart/2(EGRVlv_rGovDvt)
  EGRVlv_rOutI_mp/1 -> Limit_IPart/1(EGRVlv_rOutI_mp)

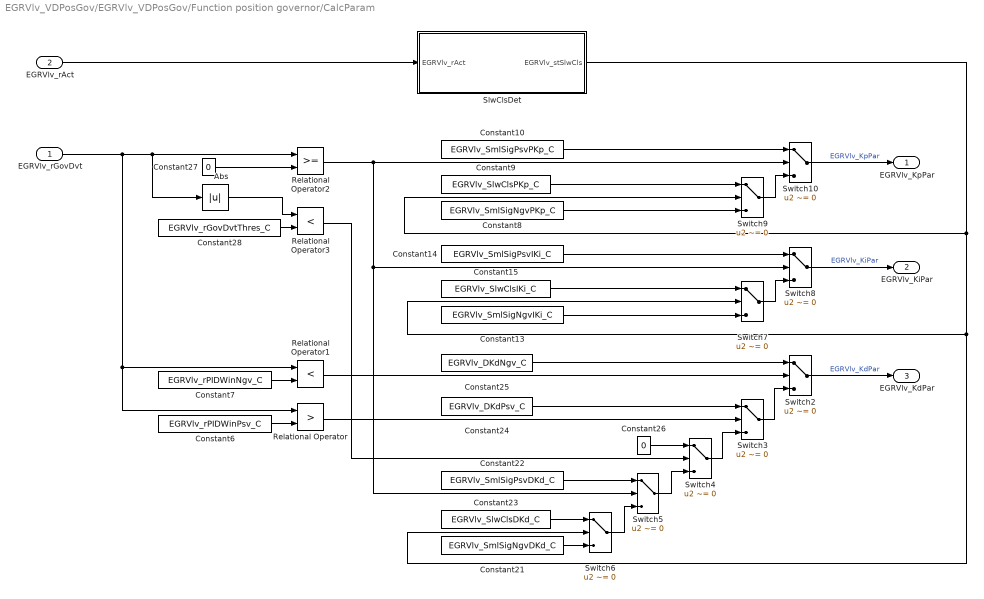
== system EGRVlv_VDPosGov/EGRVlv_VDPosGov/Function position governor/CalcParam ==
  EGRVlv_rGovDvt : Inport  Tag=%
  EGRVlv_rAct : Inport  Tag=%  Port=2
  Abs : Abs
  Constant10 : Constant  Value=EGRVlv_SmlSigPsvPKp_C
  Constant13 : Constant  Value=EGRVlv_SmlSigNgvIKi_C
  Constant14 : Constant  Value=EGRVlv_SmlSigPsvIKi_C
  Constant15 : Constant  Value=EGRVlv_SlwClsIKi_C
  Constant21 : Constant  Value=EGRVlv_SmlSigNgvDKd_C
  Constant22 : Constant  Value=EGRVlv_SmlSigPsvDKd_C
  Constant23 : Constant  Value=EGRVlv_SlwClsDKd_C
  Constant24 : Constant  Value=EGRVlv_DKdPsv_C
  Constant25 : Constant  Value=EGRVlv_DKdNgv_C
  Constant26 : Constant  Value=0  OutDataTypeStr=Inherit: Inherit via back propagation
  Constant27 : Constant  Value=0  OutDataTypeStr=Inherit: Inherit via back propagation
  Constant28 : Constant  Value=EGRVlv_rGovDvtThres_C
  Constant6 : Constant  Value=EGRVlv_rPIDWinPsv_C
  Constant7 : Constant  Value=EGRVlv_rPIDWinNgv_C
  Constant8 : Constant  Value=EGRVlv_SmlSigNgvPKp_C
  Constant9 : Constant  Value=EGRVlv_SlwClsPKp_C
  Relational Operator : RelationalOperator  Operator=>  OutDataTypeStr=boolean  RndMeth=Simplest
  Relational Operator1 : RelationalOperator  Operator=<  OutDataTypeStr=boolean  RndMeth=Simplest
  Relational Operator2 : RelationalOperator  OutDataTypeStr=boolean  RndMeth=Simplest  InputSameDT=on
  Relational Operator3 : RelationalOperator  Operator=<  OutDataTypeStr=boolean  RndMeth=Simplest
  SlwClsDet : Subsystem
  Switch{2..10} (9 alike) : Switch  Criteria=u2 ~= 0
  EGRVlv_KpPar : Outport  Tag=%
  EGRVlv_KiPar : Outport  Tag=%  Port=2
  EGRVlv_KdPar : Outport  Tag=%  Port=3
  wires:
  Constant6/1 -> Relational Operator/2
  EGRVlv_rGovDvt/1 -> Relational Operator2/1, Abs/1, Relational Operator1/1, Relational Operator/1
  Constant7/1 -> Relational Operator1/2
  Abs/1 -> Relational Operator3/1
  Constant27/1 -> Relational Operator2/2
  Constant28/1 -> Relational Operator3/2
  Relational Operator1/1 -> Switch2/2
  Constant25/1 -> Switch2/1
  Switch3/1 -> Switch2/3
  Relational Operator/1 -> Switch3/2
  Constant24/1 -> Switch3/1
  Switch4/1 -> Switch3/3
  Relational Operator3/1 -> Switch4/2
  Constant26/1 -> Switch4/1
  Switch5/1 -> Switch4/3
  Relational Operator2/1 -> Switch10/2, Switch8/2, Switch5/2
  Constant22/1 -> Switch5/1
  Switch6/1 -> Switch5/3
  Constant23/1 -> Switch6/1
  Constant21/1 -> Switch6/3
  Switch7/1 -> Switch8/3
  Constant14/1 -> Switch8/1
  Constant15/1 -> Switch7/1
  Constant13/1 -> Switch7/3
  SlwClsDet/1(EGRVlv_stSlwCls) -> Switch6/2, Switch7/2, Switch9/2
  Switch9/1 -> Switch10/3
  Constant10/1 -> Switch10/1
  Constant9/1 -> Switch9/1
  Constant8/1 -> Switch9/3
  Switch10/1 -> EGRVlv_KpPar/1  "EGRVlv_KpPar"
  Switch8/1 -> EGRVlv_KiPar/1  "EGRVlv_KiPar"
  Switch2/1 -> EGRVlv_KdPar/1  "EGRVlv_KdPar"
  EGRVlv_rAct/1 -> SlwClsDet/1(EGRVlv_rAct)

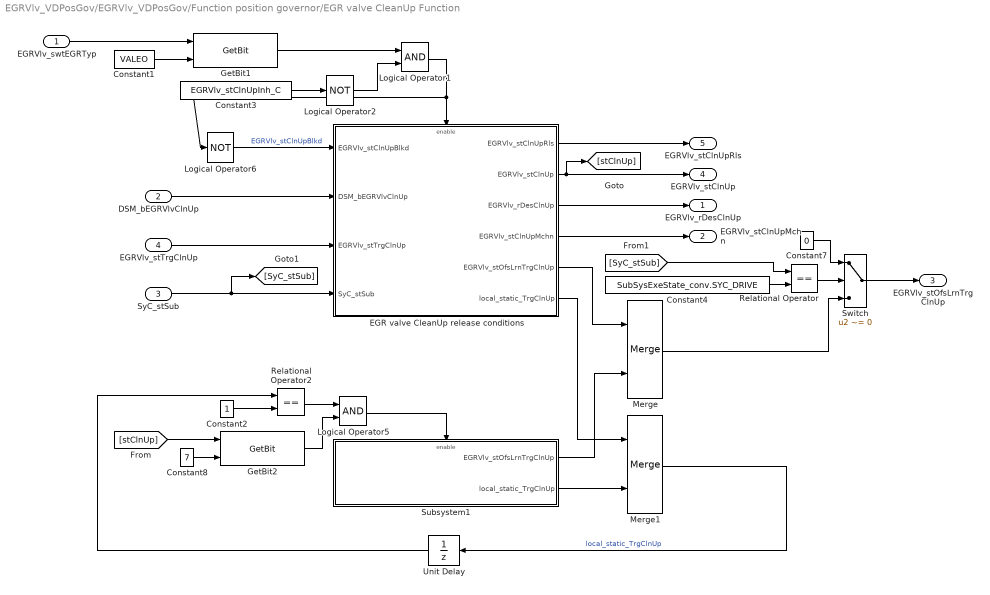
== system EGRVlv_VDPosGov/EGRVlv_VDPosGov/Function position governor/EGR valve CleanUp Function ==
  EGRVlv_swtEGRTyp : Inport  Tag=%
  DSM_bEGRVlvClnUp : Inport  Tag=%  Port=2
  SyC_stSub : Inport  Tag=%  Port=3
  EGRVlv_stTrgClnUp : Inport  Tag=%  Port=4
  Constant1 : Constant  Value=VALEO  OutDataTypeStr=uint8
  Constant2 : Constant  OutDataTypeStr=uint8
  Constant3 : Constant  Value=EGRVlv_stClnUpInh_C
  Constant4 : Constant  Value=SubSysExeState_conv.SYC_DRIVE  OutDataTypeStr=Enum:SubSysExeState_conv
  Constant7 : Constant  Value=0  OutDataTypeStr=boolean
  Constant8 : Constant  Value=7  OutDataTypeStr=uint8
  EGR valve CleanUp release conditions : Subsystem
  GetBit1 : CXLib/GetBit  dataTypeString=uint8  dataLength=0
      settings: AttributesFormatString=Get bit from %<dataTypeString>
  GetBit2 : CXLib/GetBit  dataTypeString=uint8  dataLength=0
      settings: AttributesFormatString=Get bit from %<dataTypeString>
  Logical Operator1 : Logic  AllPortsSameDT=off  OutDataTypeStr=boolean
  Logical Operator2 : Logic  Operator=NOT  AllPortsSameDT=off  OutDataTypeStr=boolean
  Logical Operator5 : Logic  AllPortsSameDT=off  OutDataTypeStr=boolean
  Logical Operator6 : Logic  Operator=NOT  AllPortsSameDT=off  OutDataTypeStr=boolean
  Merge : Merge
  Merge1 : Merge
  Relational Operator : RelationalOperator  Operator===  OutDataTypeStr=boolean  RndMeth=Simplest
  Relational Operator2 : RelationalOperator  Operator===  OutDataTypeStr=boolean  RndMeth=Simplest
  Subsystem1 : Subsystem
  Switch : Switch  Criteria=u2 ~= 0
  Unit Delay : UnitDelay  SampleTime=-1
      settings: AttributesFormatString=InitialValue=%<InitialCondition>
  EGRVlv_rDesClnUp : Outport  Tag=%
  EGRVlv_stClnUpMchn : Outport  Tag=%  Port=2
  EGRVlv_stOfsLrnTrgClnUp : Outport  Tag=%  Port=3
  EGRVlv_stClnUp : Outport  Tag=%  Port=4
  EGRVlv_stClnUpRls : Outport  Tag=%  Port=5
  wires:
  Constant1/1 -> GetBit1/2
  EGR valve CleanUp release conditions/6(local_static_TrgClnUp) -> Merge1/1
  Relational Operator2/1 -> Logical Operator5/1
  GetBit2/1 -> Logical Operator5/2
  Constant2/1 -> Relational Operator2/2
  Constant8/1 -> GetBit2/2
  EGR valve CleanUp release conditions/2(EGRVlv_stClnUp) -> [stClnUp], EGRVlv_stClnUp/1
  Merge1/1 -> Unit Delay/1  "local_static_TrgClnUp"
  Logical Operator5/1 -> Subsystem1/Enable
  Subsystem1/2(local_static_TrgClnUp) -> Merge1/2
  Subsystem1/1(EGRVlv_stOfsLrnTrgClnUp) -> Merge/2
  EGR valve CleanUp release conditions/5(EGRVlv_stOfsLrnTrgClnUp) -> Merge/1
  Unit Delay/1 -> Relational Operator2/1
  SyC_stSub/1 -> [SyC_stSub], EGR valve CleanUp release conditions/4(SyC_stSub)
  Logical Operator2/1 -> Logical Operator1/2
  Constant3/1 -> Logical Operator2/1
  GetBit1/1 -> Logical Operator1/1
  Logical Operator1/1 -> EGR valve CleanUp release conditions/Enable, Logical Operator6/1
  Constant4/1 -> Relational Operator/2
  Relational Operator/1 -> Switch/2
  Merge/1 -> Switch/3
  Switch/1 -> EGRVlv_stOfsLrnTrgClnUp/1
  Constant7/1 -> Switch/1
  [SyC_stSub] -> Relational Operator/1
  Logical Operator6/1 -> EGR valve CleanUp release conditions/1(EGRVlv_stClnUpBlkd)  "EGRVlv_stClnUpBlkd"
  DSM_bEGRVlvClnUp/1 -> EGR valve CleanUp release conditions/2(DSM_bEGRVlvClnUp)
  EGRVlv_stTrgClnUp/1 -> EGR valve CleanUp release conditions/3(EGRVlv_stTrgClnUp)
  EGRVlv_swtEGRTyp/1 -> GetBit1/1
  [stClnUp] -> GetBit2/1
  EGR valve CleanUp release conditions/1(EGRVlv_stClnUpRls) -> EGRVlv_stClnUpRls/1
  EGR valve CleanUp release conditions/3(EGRVlv_rDesClnUp) -> EGRVlv_rDesClnUp/1
  EGR valve CleanUp release conditions/4(EGRVlv_stClnUpMchn) -> EGRVlv_stClnUpMchn/1

== system EGRVlv_VDPosGov/EGRVlv_VDPosGov/Function position governor/I_comp ==
  note: %sampletime(us)%
  note: %1/s,resolution=2^15%
  Dvt : Inport
  T0 : Inport  Port=2  OutDataTypeStr=uint32
  Ki : Inport  Port=3
  KiPos : Inport  Port=4
  KiNeg : Inport  Port=5
  WinPos : Inport  Port=6
  WinNeg : Inport  Port=7
  stInit : Inport  Port=8  OutDataTypeStr=boolean
  InitVal : Inport  Port=9
  Calc : Subsystem
  Chart : CXLib/I_S16/Chart
  Data Store Memory : DataStoreMemory  DataStoreName=outputlast1  ReadBeforeWriteMsg=warning  WriteAfterWriteMsg=warning  WriteAfterReadMsg=warning  ShowAdditionalParam=off  OutDataTypeStr=fixdt(1,32,2^-16,0)
  Init : Subsystem
  Switch1 : Switch  Criteria=u2 ~= 0  SaturateOnIntegerOverflow=on  InputSameDT=on
  Out : Outport
  wires:
  Chart/1 -> Init/Trigger
  stInit/1 -> Chart/1, Switch1/2
  Ki/1 -> Calc/3(Ki)
  Dvt/1 -> Calc/1(Dvt)
  T0/1 -> Calc/2(T0)
  Calc/1(Out) -> Switch1/3
  KiNeg/1 -> Calc/5(KiNeg)
  Switch1/1 -> Out/1
  Chart/2 -> Calc/Trigger
  WinNeg/1 -> Calc/7(WinNeg)
  InitVal/1 -> Init/1(InitVal), Switch1/1
  WinPos/1 -> Calc/6(WinPos)
  KiPos/1 -> Calc/4(KiPos)

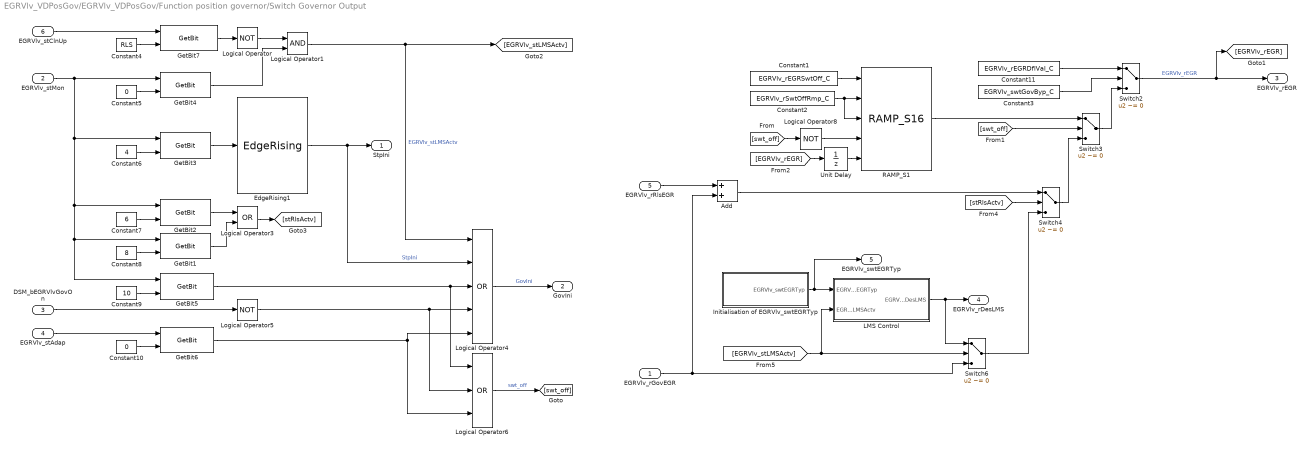
== system EGRVlv_VDPosGov/EGRVlv_VDPosGov/Function position governor/Switch Governor Output ==
  EGRVlv_rGovEGR : Inport  Tag=%
  EGRVlv_stMon : Inport  Tag=%  Port=2
  DSM_bEGRVlvGovOn : Inport  Tag=%  Port=3
  EGRVlv_stAdap : Inport  Tag=%  Port=4
  EGRVlv_rRlsEGR : Inport  Tag=%  Port=5
  EGRVlv_stClnUp : Inport  Tag=%  Port=6
  Add : Sum  SaturateOnIntegerOverflow=on
  Constant1 : Constant  Value=EGRVlv_rEGRSwtOff_C
  Constant10 : Constant  Value=0  OutDataTypeStr=uint8
  Constant11 : Constant  Value=EGRVlv_rEGRDflVal_C
  Constant2 : Constant  Value=EGRVlv_rSwtOffRmp_C
  Constant3 : Constant  Value=EGRVlv_swtGovByp_C
  Constant4 : Constant  Value=RLS
  Constant5 : Constant  Value=0  OutDataTypeStr=uint8
  Constant6 : Constant  Value=4  OutDataTypeStr=uint8
  Constant7 : Constant  Value=6  OutDataTypeStr=uint8
  Constant8 : Constant  Value=8  OutDataTypeStr=uint8
  Constant9 : Constant  Value=10  OutDataTypeStr=uint8
  EdgeRising1 : CXLib/EdgeRising
  GetBit{1..6} (6 alike) : CXLib/GetBit  dataTypeString=uint16  dataLength=0
      settings: AttributesFormatString=Get bit from %<dataTypeString>
  GetBit7 : CXLib/GetBit  dataTypeString=uint8  dataLength=0
      settings: AttributesFormatString=Get bit from %<dataTypeString>
  Initialisation of EGRVlv_swtEGRTyp : Subsystem
  LMS Control : Subsystem
  Logical Operator : Logic  Operator=NOT  AllPortsSameDT=off  OutDataTypeStr=boolean
  Logical Operator1 : Logic  AllPortsSameDT=off  OutDataTypeStr=boolean
  Logical Operator3 : Logic  Operator=OR  AllPortsSameDT=off  OutDataTypeStr=boolean
  Logical Operator4 : Logic  Operator=OR  Inputs=5  AllPortsSameDT=off  OutDataTypeStr=boolean
  Logical Operator5 : Logic  Operator=NOT  AllPortsSameDT=off  OutDataTypeStr=boolean
  Logical Operator6 : Logic  Operator=OR  Inputs=3  AllPortsSameDT=off  OutDataTypeStr=boolean
  Logical Operator8 : Logic  Operator=NOT  AllPortsSameDT=off  OutDataTypeStr=boolean
  RAMP_S1 : CXLib/RAMP_S16
  Switch{2..4,6} (4 alike) : Switch  Criteria=u2 ~= 0
  Unit Delay : UnitDelay  SampleTime=-1
      settings: AttributesFormatString=InitialValue=%<InitialCondition>
  StpIni : Outport  Tag=%
  GovIni : Outport  Tag=%  Port=2
  EGRVlv_rEGR : Outport  Tag=%  Port=3
  EGRVlv_rDesLMS : Outport  Tag=%  Port=4
  EGRVlv_swtEGRTyp : Outport  Tag=%  Port=5
  wires:
  Logical Operator4/1 -> GovIni/1  "GovIni"
  Logical Operator/1 -> Logical Operator1/1
  Logical Operator5/1 -> Logical Operator4/4, Logical Operator6/2
  DSM_bEGRVlvGovOn/1 -> Logical Operator5/1
  EdgeRising1/1 -> Logical Operator4/2, StpIni/1  "StpIni"
  Logical Operator6/1 -> [swt_off]  "swt_off"
  Logical Operator1/1 -> [EGRVlv_stLMSActv], Logical Operator4/1  "EGRVlv_stLMSActv"
  EGRVlv_rRlsEGR/1 -> Add/1
  EGRVlv_rGovEGR/1 -> Add/2, Switch6/3
  Switch2/1 -> EGRVlv_rEGR/1, [EGRVlv_rEGR]  "EGRVlv_rEGR"
  Constant2/1 -> RAMP_S1/3, RAMP_S1/2
  Initialisation of EGRVlv_swtEGRTyp/1(EGRVlv_swtEGRTyp) -> EGRVlv_swtEGRTyp/1, LMS Control/1(EGRVlv_swtEGRTyp)
  LMS Control/1(EGRVlv_rDesLMS) -> EGRVlv_rDesLMS/1, Switch6/1
  Switch3/1 -> Switch2/3
  Switch4/1 -> Switch3/3
  Switch6/1 -> Switch4/3
  Constant11/1 -> Switch2/1
  Constant3/1 -> Switch2/2
  [swt_off] -> Switch3/2
  RAMP_S1/1 -> Switch3/1
  [EGRVlv_rEGR] -> Unit Delay/1
  Logical Operator3/1 -> [stRlsActv]
  [EGRVlv_stLMSActv] -> Switch6/2, LMS Control/2(EGRVlv_stLMSActv)
  [swt_off] -> Logical Operator8/1
  Logical Operator8/1 -> RAMP_S1/4
  GetBit7/1 -> Logical Operator/1
  GetBit4/1 -> Logical Operator1/2
  GetBit3/1 -> EdgeRising1/1
  GetBit2/1 -> Logical Operator3/1
  GetBit1/1 -> Logical Operator3/2
  GetBit5/1 -> Logical Operator6/1, Logical Operator4/3
  GetBit6/1 -> Logical Operator4/5, Logical Operator6/3
  Constant5/1 -> GetBit4/2
  Constant6/1 -> GetBit3/2
  Constant7/1 -> GetBit2/2
  Constant8/1 -> GetBit1/2
  Constant9/1 -> GetBit5/2
  Constant10/1 -> GetBit6/2
  Constant4/1 -> GetBit7/2
  EGRVlv_stMon/1 -> GetBit4/1, GetBit3/1, GetBit2/1, GetBit1/1, GetBit5/1
  Unit Delay/1 -> RAMP_S1/5
  Constant1/1 -> RAMP_S1/1
  EGRVlv_stClnUp/1 -> GetBit7/1
  EGRVlv_stAdap/1 -> GetBit6/1
  [stRlsActv] -> Switch4/2
  Add/1 -> Switch4/1

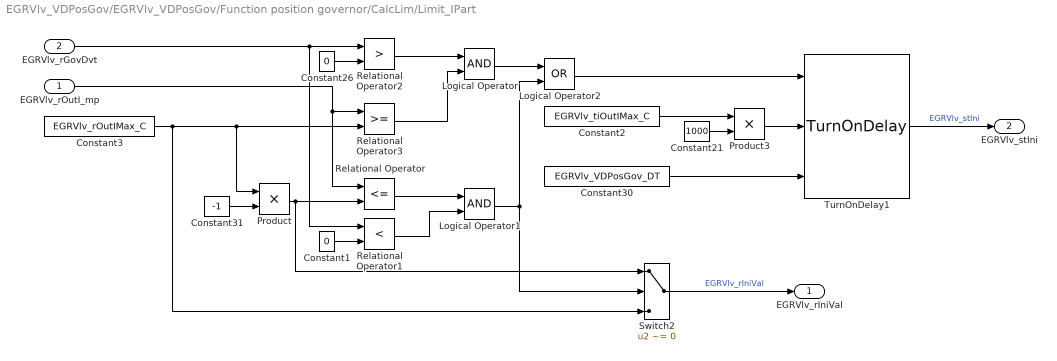
== system EGRVlv_VDPosGov/EGRVlv_VDPosGov/Function position governor/CalcLim/Limit_IPart ==
  EGRVlv_rOutI_mp : Inport  Tag=%
  EGRVlv_rGovDvt : Inport  Tag=%  Port=2
  Constant1 : Constant  Value=0  OutDataTypeStr=Inherit: Inherit via back propagation
  Constant2 : Constant  Value=EGRVlv_tiOutIMax_C
  Constant21 : Constant  Value=1000  OutDataTypeStr=uint16
  Constant26 : Constant  Value=0  OutDataTypeStr=Inherit: Inherit via back propagation
  Constant3 : Constant  Value=EGRVlv_rOutIMax_C
  Constant30 : Constant  Value=EGRVlv_VDPosGov_DT
  Constant31 : Constant  Value=-1  OutDataTypeStr=int8
  Logical Operator : Logic  AllPortsSameDT=off  OutDataTypeStr=boolean
  Logical Operator1 : Logic  AllPortsSameDT=off  OutDataTypeStr=boolean
  Logical Operator2 : Logic  Operator=OR  AllPortsSameDT=off  OutDataTypeStr=boolean
  Product : Product  OutDataTypeStr=Prc_100_rate  SaturateOnIntegerOverflow=on
  Product3 : Product  OutDataTypeStr=uint32  SaturateOnIntegerOverflow=on
  Relational Operator : RelationalOperator  Operator=<=  OutDataTypeStr=boolean  RndMeth=Simplest
  Relational Operator1 : RelationalOperator  Operator=<  OutDataTypeStr=boolean  RndMeth=Simplest  InputSameDT=on
  Relational Operator2 : RelationalOperator  Operator=>  OutDataTypeStr=boolean  RndMeth=Simplest  InputSameDT=on
  Relational Operator3 : RelationalOperator  OutDataTypeStr=boolean  RndMeth=Simplest
  Switch2 : Switch  Criteria=u2 ~= 0
  TurnOnDelay1 : CXLib/TurnOnDelay
  EGRVlv_rIniVal : Outport  Tag=%
  EGRVlv_stIni : Outport  Tag=%  Port=2
  wires:
  Constant31/1 -> Product/2
  Constant30/1 -> TurnOnDelay1/3
  Relational Operator1/1 -> Logical Operator1/2
  EGRVlv_rGovDvt/1 -> Relational Operator2/1, Relational Operator1/1
  Constant26/1 -> Relational Operator2/2
  Relational Operator/1 -> Logical Operator1/1
  Constant1/1 -> Relational Operator1/2
  Logical Operator/1 -> Logical Operator2/1
  Relational Operator3/1 -> Logical Operator/2
  Constant2/1 -> Product3/1
  Relational Operator2/1 -> Logical Operator/1
  Logical Operator2/1 -> TurnOnDelay1/1
  EGRVlv_rOutI_mp/1 -> Relational Operator3/1, Relational Operator/1
  Product3/1 -> TurnOnDelay1/2
  Constant21/1 -> Product3/2
  TurnOnDelay1/1 -> EGRVlv_stIni/1  "EGRVlv_stIni"
  Product/1 -> Switch2/1, Relational Operator/2
  Logical Operator1/1 -> Logical Operator2/2, Switch2/2
  Constant3/1 -> Switch2/3, Product/1, Relational Operator3/2
  Switch2/1 -> EGRVlv_rIniVal/1  "EGRVlv_rIniVal"

== system EGRVlv_VDPosGov/EGRVlv_VDPosGov/Function position governor/CalcParam/SlwClsDet ==
  EGRVlv_rAct : Inport  Tag=%
  Constant1 : Constant  Value=EGRVlv_tiParDT1_C
  Constant2 : Constant  Value=0  OutDataTypeStr=Inherit: Inherit via back propagation
  Constant21 : Constant  Value=1000  OutDataTypeStr=uint16
  Constant27 : Constant  Value=false  OutDataTypeStr=boolean
  Constant29 : Constant  Value=EGRVlv_KdParDT1_C
  Constant3 : Constant  Value=0  OutDataTypeStr=Inherit: Inherit via back propagation
  Constant30 : Constant  Value=EGRVlv_VDPosGov_DT
  Constant31 : Constant  Value=-1  OutDataTypeStr=int8
  Constant32 : Constant  Value=EGRVlv_drActNgv_C
  Constant33 : Constant  Value=EGRVlv_rActNgv_C
  Constant4 : Constant  Value=1000  OutDataTypeStr=uint16
  DT1_S16 : CXLib/DT1_S16
  Logical Operator : Logic  AllPortsSameDT=off  OutDataTypeStr=boolean
  Product : Product  OutDataTypeStr=DutyCycle_rate_s  SaturateOnIntegerOverflow=on
  Product1 : Product  OutDataTypeStr=uint32  SaturateOnIntegerOverflow=on
  Product3 : Product  OutDataTypeStr=uint32  SaturateOnIntegerOverflow=on
  Relational Operator4 : RelationalOperator  Operator=>  OutDataTypeStr=boolean  RndMeth=Simplest
  Relational Operator5 : RelationalOperator  Operator=<  OutDataTypeStr=boolean  RndMeth=Simplest
  EGRVlv_stSlwCls : Outport  Tag=%
  wires:
  DT1_S16/1 -> Product/1
  Constant31/1 -> Product/2
  Relational Operator4/1 -> Logical Operator/1
  Relational Operator5/1 -> Logical Operator/2
  Constant32/1 -> Relational Operator4/2
  Constant2/1 -> DT1_S16/2
  Constant3/1 -> DT1_S16/3
  Constant27/1 -> DT1_S16/1
  Product/1 -> Relational Operator4/1  "EGRVlv_drAct_mp"
  Constant29/1 -> DT1_S16/7
  Logical Operator/1 -> EGRVlv_stSlwCls/1  "EGRVlv_stSlwCls"
  EGRVlv_rAct/1 -> DT1_S16/6, Relational Operator5/1
  Constant33/1 -> Relational Operator5/2
  Constant21/1 -> Product3/2
  Product3/1 -> DT1_S16/4
  Constant30/1 -> Product3/1
  Constant4/1 -> Product1/2
  Product1/1 -> DT1_S16/5
  Constant1/1 -> Product1/1
